simulink model "SimulinkEKF1"  (R2013b)
settings: Solver=ode3  StartTime=0.0  StopTime=20  RelTol=1e-3
undefined symbols (not defined in the file): Ad, Bd
settings Model: Creator=ThiagoCordeiro  LastModifiedBy=ThiagoFelippe

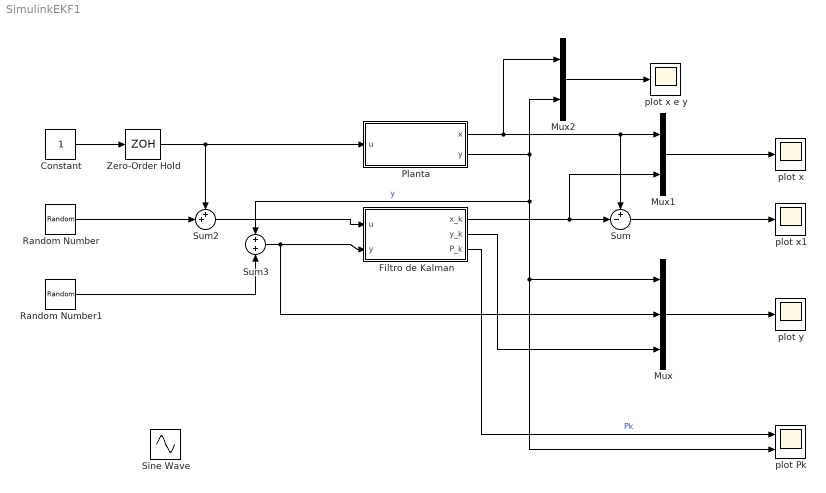
== system SimulinkEKF1 ==
  Constant : Constant
  Filtro de Kalman : Subsystem
  Mux : Mux  Inputs=3
  Mux1 : Mux  Inputs=2
  Mux2 : Mux  Inputs=2
  Planta : Subsystem
  Random Number : RandomNumber  Seed=round(rand(1)*(2^32-1))  SampleTime=0.01
  Random Number1 : RandomNumber  Seed=round(rand(1)*(2^32-1))  SampleTime=0.01
  Sine Wave : Sin  Amplitude=2  Phase=pi/2  SampleTime=0
  Sum : Sum  Inputs=+-|
  Sum2 : Sum  Inputs=++|
  Sum3 : Sum  Inputs=+|+
  Zero-Order Hold : ZeroOrderHold  SampleTime=0.01
  plot Pk : Scope  NumInputPorts=2
      settings: ShowLegends=on  YMin=-5~-5  YMax=5~5  SaveName=ScopeData4
  plot x : Scope
  plot x e y : Scope
      settings: SaveName=ScopeData6
  plot x1 : Scope
  plot y : Scope
      settings: ShowLegends=on  SaveName=ScopeData2
  wires:
  Mux/1 -> plot y/1
  Zero-Order Hold/1 -> Planta/1(u), Sum2/1
  Random Number/1 -> Sum2/2
  Random Number1/1 -> Sum3/2
  Constant/1 -> Zero-Order Hold/1
  Sum2/1 -> Filtro de Kalman/1(u)
  Sum3/1 -> Mux/2, Filtro de Kalman/2(y)
  Planta/2(y) -> plot Pk/2, Mux/1, Sum3/1, Mux2/2  "y"
  Planta/1(x) -> Mux2/1, Sum/1, Mux1/1
  Filtro de Kalman/1(x_k) -> Sum/2, Mux1/2
  Mux1/1 -> plot x/1
  Filtro de Kalman/2(y_k) -> Mux/3
  Sum/1 -> plot x1/1
  Filtro de Kalman/3(P_k) -> plot Pk/1  "Pk"
  Mux2/1 -> plot x e y/1

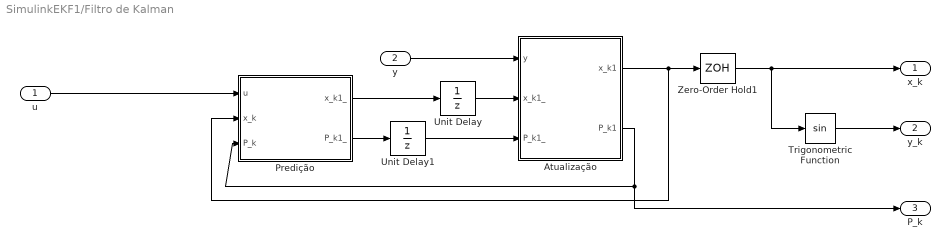
== system SimulinkEKF1/Filtro de Kalman ==
  u : Inport
  y : Inport  Port=2
  Atualização : Subsystem
  Predição : Subsystem
  Trigonometric Function : Trigonometry
  Unit Delay : UnitDelay  InitialCondition=randn(1)  SampleTime=0.01
  Unit Delay1 : UnitDelay  InitialCondition=1  SampleTime=0.01
  Zero-Order Hold1 : ZeroOrderHold  SampleTime=0.01
  x_k : Outport
  y_k : Outport  Port=2
  P_k : Outport  Port=3
  wires:
  u/1 -> Predição/1(u)
  y/1 -> Atualização/1(y)
  Atualização/1(x_k1) -> Predição/2(x_k), Zero-Order Hold1/1
  Atualização/2(P_k1) -> P_k/1, Predição/3(P_k)
  Predição/2(P_k1_) -> Unit Delay1/1
  Unit Delay1/1 -> Atualização/3(P_k1_)
  Unit Delay/1 -> Atualização/2(x_k1_)
  Predição/1(x_k1_) -> Unit Delay/1
  Zero-Order Hold1/1 -> Trigonometric Function/1, x_k/1
  Trigonometric Function/1 -> y_k/1

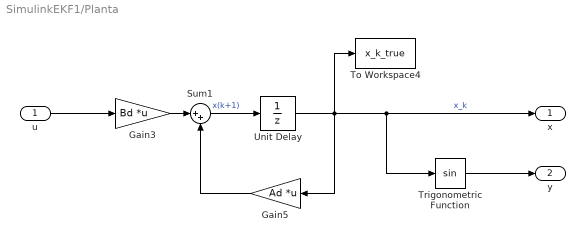
== system SimulinkEKF1/Planta ==
  u : Inport
  Gain3 : Gain  Gain=Bd  Multiplication=Matrix(K*u)
  Gain5 : Gain  Gain=Ad  Multiplication=Matrix(K*u)
  Sum1 : Sum  Inputs=|++
  To Workspace4 : ToWorkspace  VariableName=x_k_true  SampleTime=-1  SaveFormat=Timeseries
  Trigonometric Function : Trigonometry
  Unit Delay : UnitDelay  InitialCondition=[0]  SampleTime=-1
  x : Outport
  y : Outport  Port=2
  wires:
  Gain3/1 -> Sum1/1
  Sum1/1 -> Unit Delay/1  "x(k+1)"
  Unit Delay/1 -> Trigonometric Function/1, x/1, To Workspace4/1, Gain5/1  "x_k"
  Gain5/1 -> Sum1/2
  u/1 -> Gain3/1
  Trigonometric Function/1 -> y/1

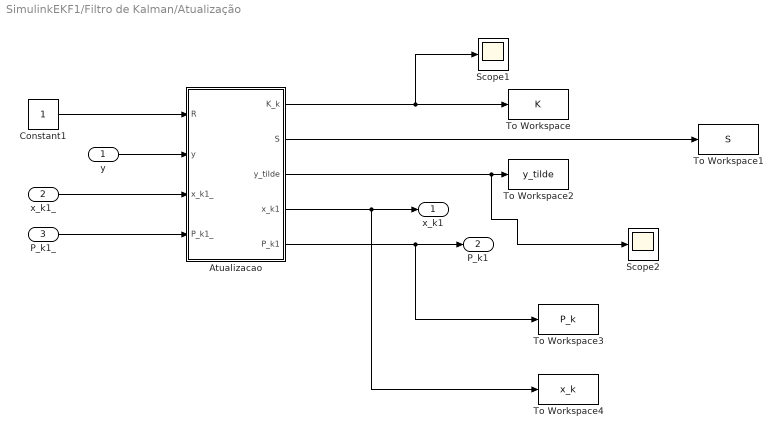
== system SimulinkEKF1/Filtro de Kalman/Atualização ==
  y : Inport
  x_k1_ : Inport  Port=2
  P_k1_ : Inport  Port=3
  Atualizacao : MATLAB Function  TreatAsAtomicUnit=on  SystemSampleTime=0.01
  Constant1 : Constant
  Scope1 : Scope
      settings: SaveName=ScopeData3
  Scope2 : Scope
      settings: SaveName=ScopeData5
  To Workspace : ToWorkspace  VariableName=K  SampleTime=-1  SaveFormat=Timeseries
  To Workspace1 : ToWorkspace  VariableName=S  SampleTime=-1  SaveFormat=Timeseries
  To Workspace2 : ToWorkspace  VariableName=y_tilde  SampleTime=-1  SaveFormat=Timeseries
  To Workspace3 : ToWorkspace  VariableName=P_k  SampleTime=-1  SaveFormat=Timeseries
  To Workspace4 : ToWorkspace  VariableName=x_k  SampleTime=-1  SaveFormat=Timeseries
  x_k1 : Outport
  P_k1 : Outport  Port=2
  wires:
  y/1 -> Atualizacao/2(y)
  x_k1_/1 -> Atualizacao/3(x_k1_)
  P_k1_/1 -> Atualizacao/4(P_k1_)
  Atualizacao/4(x_k1) -> To Workspace4/1, x_k1/1
  Atualizacao/5(P_k1) -> To Workspace3/1, P_k1/1
  Constant1/1 -> Atualizacao/1(R)
  Atualizacao/1(K_k) -> Scope1/1, To Workspace/1
  Atualizacao/2(S) -> To Workspace1/1
  Atualizacao/3(y_tilde) -> Scope2/1, To Workspace2/1

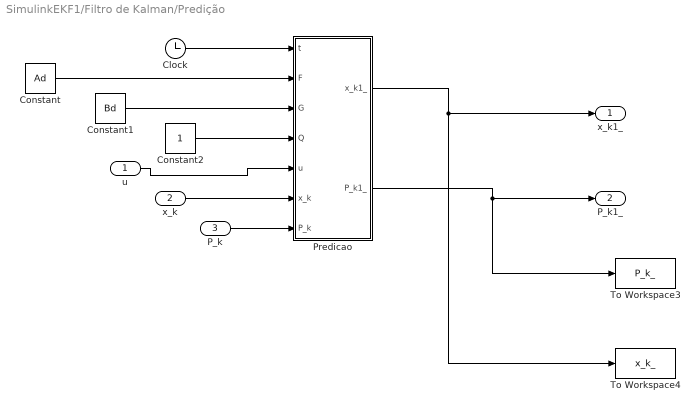
== system SimulinkEKF1/Filtro de Kalman/Predição ==
  u : Inport
  x_k : Inport  Port=2
  P_k : Inport  Port=3
  Clock : Clock
  Constant : Constant  Value=Ad
  Constant1 : Constant  Value=Bd  VectorParams1D=off
  Constant2 : Constant
  Predicao : MATLAB Function  TreatAsAtomicUnit=on  SystemSampleTime=0.01
  To Workspace3 : ToWorkspace  VariableName=P_k_  SampleTime=-1  SaveFormat=Timeseries
  To Workspace4 : ToWorkspace  VariableName=x_k_  SampleTime=-1  SaveFormat=Timeseries
  x_k1_ : Outport
  P_k1_ : Outport  Port=2
  wires:
  u/1 -> Predicao/5(u)
  x_k/1 -> Predicao/6(x_k)
  P_k/1 -> Predicao/7(P_k)
  Constant/1 -> Predicao/2(F)
  Constant1/1 -> Predicao/3(G)
  Constant2/1 -> Predicao/4(Q)
  Predicao/1(x_k1_) -> To Workspace4/1, x_k1_/1
  Predicao/2(P_k1_) -> To Workspace3/1, P_k1_/1
  Clock/1 -> Predicao/1(t)

== matlab function SimulinkEKF1/Filtro de Kalman/Atualização/Atualizacao ==
  data: R input; K_k output; S output; y_tilde output; y input; x_k1_ input; P_k1_ input; x_k1 output; P_k1 output
function [K_k, S, y_tilde, x_k1, P_k1] = fcn(R, y, x_k1_, P_k1_)
%#codegen

y_hat = sin(x_k1_);
H = cos(x_k1_);

S = H * P_k1_ * H' + R;
Pxy = P_k1_ * H';
K_k  =  Pxy / S;
KH = K_k*H;
I = eye(size(KH));
I_KH = I - KH;
P_k1 = I_KH * P_k1_ * I_KH' + K_k * R * K_k';


y_tilde = y - y_hat;
x_k1 = x_k1_ + K_k * y_tilde;

== matlab function SimulinkEKF1/Filtro de Kalman/Predição/Predicao ==
  data: t input; F input; G input; Q input; u input; x_k1_ output; x_k input; P_k input; P_k1_ output
function [x_k1_,P_k1_] = fcn(t, F, G, Q, u, x_k, P_k)
%#codegen
if t >= 0
    x_k1_ = F*x_k + G*u;
    P_k1_ = F*P_k*F' + G*Q*G';
else
    x_k1_ = x_k;
    P_k1_ = P_k;
end
